simulink subsystem "matteEnergyBalance"  (R2024a)
settings: Solver=VariableStepAuto  StartTime=0.0  StopTime=3600*24  RelTol=1e-3
undefined symbols (not defined in the file): air_specific_heat_capacity, bath_area, matte_specific_heat_capacity, slag_matte_heat_transfer_coefficient
settings Model: DataDictionary=constants.sldd  EnableAccessToBaseWorkspace=off  DefaultTestHarness=matteEnergyBalance_Harness_Constants  Creator=eunice.duplessis  LastModifiedBy=jason.miskin

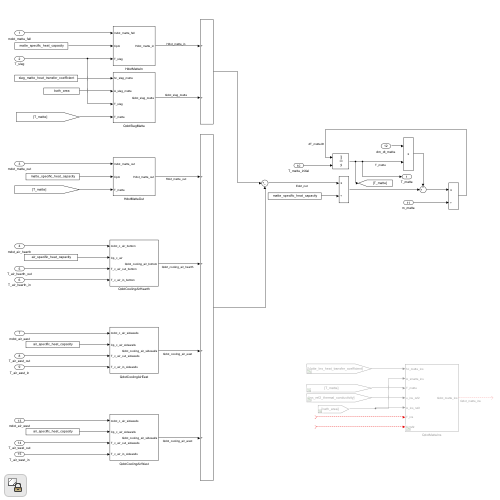
[thumbnail: Simulink's stored preview of the top-level diagram]
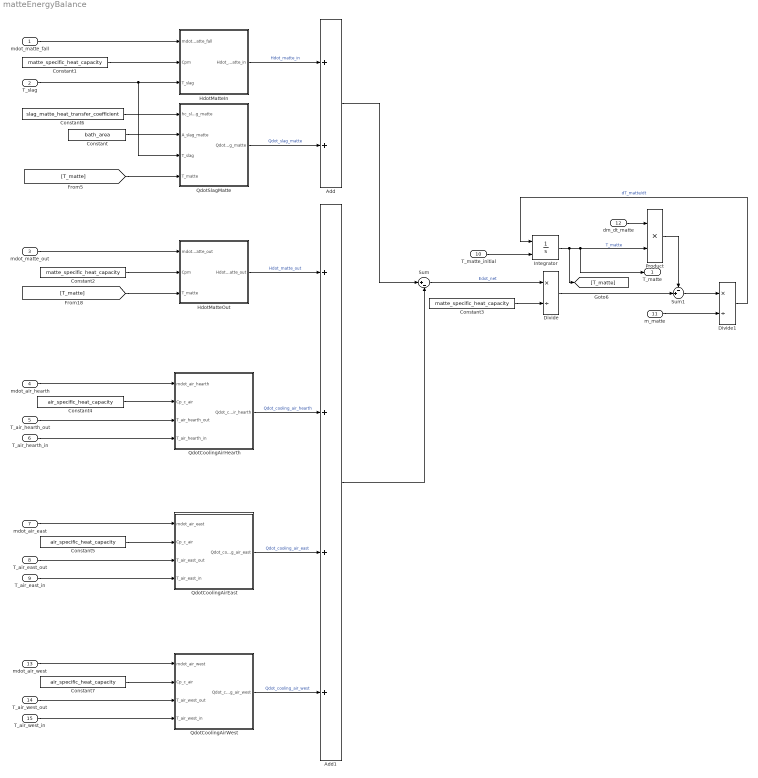
== system matteEnergyBalance ==
  mdot_matte_fall : Inport
  T_slag : Inport  Port=2
  mdot_matte_out : Inport  Port=3
  mdot_air_hearth : Inport  Port=4
  T_air_hearth_out : Inport  Port=5
  T_air_hearth_in : Inport  Port=6
  mdot_air_east : Inport  Port=7
  T_air_east_out : Inport  Port=8
  T_air_east_in : Inport  Port=9
  T_matte_initial : Inport  Port=10
  m_matte : Inport  Port=11
  dm_dt_matte : Inport  Port=12
  mdot_air_west : Inport  Port=13
  T_air_west_out : Inport  Port=14
  T_air_west_in : Inport  Port=15
  Add : Sum  Inputs=2
  Add1 : Sum  Inputs=4
  Constant : Constant  Value=bath_area
  Constant1 : Constant  Value=matte_specific_heat_capacity
  Constant2 : Constant  Value=matte_specific_heat_capacity
  Constant3 : Constant  Value=matte_specific_heat_capacity
  Constant4 : Constant  Value=air_specific_heat_capacity
  Constant5 : Constant  Value=air_specific_heat_capacity
  Constant6 : Constant  Value=slag_matte_heat_transfer_coefficient
  Constant7 : Constant  Value=air_specific_heat_capacity
  Divide : Product  Inputs=*/
  Divide1 : Product  Inputs=*/
  HdotMatteIn : Subsystem
  HdotMatteOut : Subsystem
  Integrator : Integrator  InitialConditionSource=external
  Product : Product
  QdotCoolingAirEast : Subsystem
  QdotCoolingAirHearth : Subsystem
  QdotCoolingAirWest : Subsystem
  QdotSlagMatte : Subsystem
  Sum : Sum  Inputs=|+-
  Sum1 : Sum  Inputs=-+|
  T_matte : Outport
  wires:
  Sum/1 -> Divide/1  "Edot_net"
  T_slag/1 -> QdotSlagMatte/3(T_slag), HdotMatteIn/3(T_slag)
  m_matte/1 -> Divide1/2
  [T_matte] -> QdotSlagMatte/4(T_matte)
  Product/1 -> Sum1/1
  dm_dt_matte/1 -> Product/1
  HdotMatteIn/1(Hdot_matte_in) -> Add/1  "Hdot_matte_in"
  Add/1 -> Sum/1
  Divide/1 -> Sum1/2
  Divide1/1 -> Integrator/1  "dT_matte/dt"
  Constant/1 -> QdotSlagMatte/2(A_slag_matte)
  Constant2/1 -> HdotMatteOut/2(Cpm)
  T_matte_initial/1 -> Integrator/2
  Integrator/1 -> [T_matte], T_matte/1, Product/2  "T_matte"
  HdotMatteOut/1(Hdot_matte_out) -> Add1/1  "Hdot_matte_out"
  mdot_air_east/1 -> QdotCoolingAirEast/1(mdot_air_east)
  mdot_matte_out/1 -> HdotMatteOut/1(mdot_matte_out)
  Sum1/1 -> Divide1/1
  QdotCoolingAirEast/1(Qdot_cooling_air_east) -> Add1/3  "Qdot_cooling_air_east"
  Constant6/1 -> QdotSlagMatte/1(hc_slag_matte)
  QdotSlagMatte/1(Qdot_slag_matte) -> Add/2  "Qdot_slag_matte"
  Constant3/1 -> Divide/2
  Constant1/1 -> HdotMatteIn/2(Cpm)
  Add1/1 -> Sum/2
  [T_matte] -> HdotMatteOut/3(T_matte)
  mdot_matte_fall/1 -> HdotMatteIn/1(mdot_matte_fall)
  Constant5/1 -> QdotCoolingAirEast/2(Cp_c_air)
  T_air_east_out/1 -> QdotCoolingAirEast/3(T_air_east_out)
  T_air_east_in/1 -> QdotCoolingAirEast/4(T_air_east_in)
  T_air_hearth_in/1 -> QdotCoolingAirHearth/4(T_air_hearth_in)
  Constant4/1 -> QdotCoolingAirHearth/2(Cp_c_air)
  QdotCoolingAirHearth/1(Qdot_cooling_air_hearth) -> Add1/2  "Qdot_cooling_air_hearth"
  mdot_air_hearth/1 -> QdotCoolingAirHearth/1(mdot_air_hearth)
  T_air_hearth_out/1 -> QdotCoolingAirHearth/3(T_air_hearth_out)
  T_air_west_in/1 -> QdotCoolingAirWest/4(T_air_west_in)
  T_air_west_out/1 -> QdotCoolingAirWest/3(T_air_west_out)
  Constant7/1 -> QdotCoolingAirWest/2(Cp_c_air)
  QdotCoolingAirWest/1(Qdot_cooling_air_west) -> Add1/4  "Qdot_cooling_air_west"
  mdot_air_west/1 -> QdotCoolingAirWest/1(mdot_air_west)

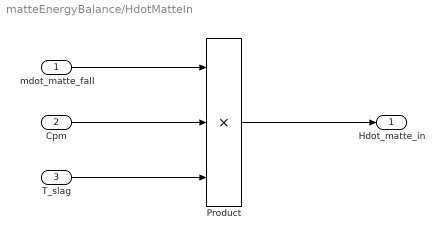
== system matteEnergyBalance/HdotMatteIn ==
  mdot_matte_fall : Inport
  Cpm : Inport  Port=2
  T_slag : Inport  Port=3
  Product : Product  Inputs=3
  Hdot_matte_in : Outport
  wires:
  T_slag/1 -> Product/3
  mdot_matte_fall/1 -> Product/1
  Product/1 -> Hdot_matte_in/1
  Cpm/1 -> Product/2

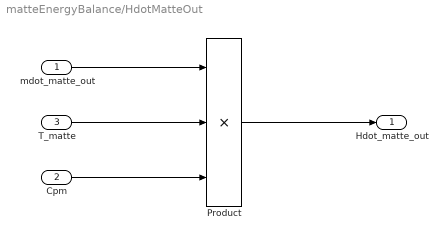
== system matteEnergyBalance/HdotMatteOut ==
  mdot_matte_out : Inport
  Cpm : Inport  Port=2
  T_matte : Inport  Port=3
  Product : Product  Inputs=3
  Hdot_matte_out : Outport
  wires:
  Cpm/1 -> Product/3
  mdot_matte_out/1 -> Product/1
  T_matte/1 -> Product/2
  Product/1 -> Hdot_matte_out/1

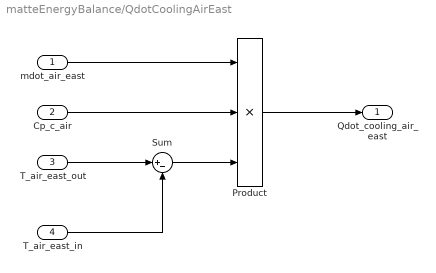
== system matteEnergyBalance/QdotCoolingAirEast ==
  mdot_air_east : Inport
  Cp_c_air : Inport  Port=2
  T_air_east_out : Inport  Port=3
  T_air_east_in : Inport  Port=4
  Product : Product  Inputs=3
  Sum : Sum  Inputs=|+-
  Qdot_cooling_air_east : Outport
  wires:
  mdot_air_east/1 -> Product/1
  T_air_east_out/1 -> Sum/1
  T_air_east_in/1 -> Sum/2
  Sum/1 -> Product/3
  Cp_c_air/1 -> Product/2
  Product/1 -> Qdot_cooling_air_east/1

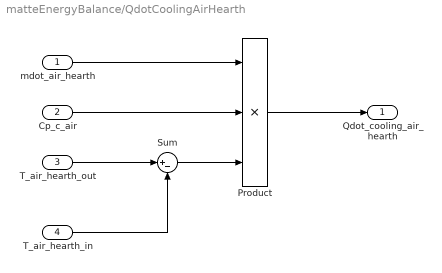
== system matteEnergyBalance/QdotCoolingAirHearth ==
  mdot_air_hearth : Inport
  Cp_c_air : Inport  Port=2
  T_air_hearth_out : Inport  Port=3
  T_air_hearth_in : Inport  Port=4
  Product : Product  Inputs=3
  Sum : Sum  Inputs=|+-
  Qdot_cooling_air_hearth : Outport
  wires:
  mdot_air_hearth/1 -> Product/1
  T_air_hearth_out/1 -> Sum/1
  T_air_hearth_in/1 -> Sum/2
  Sum/1 -> Product/3
  Cp_c_air/1 -> Product/2
  Product/1 -> Qdot_cooling_air_hearth/1

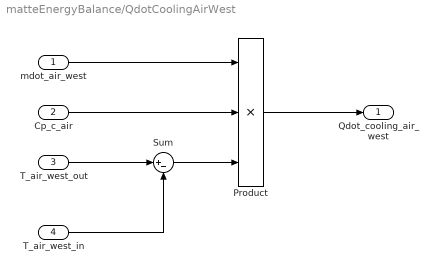
== system matteEnergyBalance/QdotCoolingAirWest ==
  mdot_air_west : Inport
  Cp_c_air : Inport  Port=2
  T_air_west_out : Inport  Port=3
  T_air_west_in : Inport  Port=4
  Product : Product  Inputs=3
  Sum : Sum  Inputs=|+-
  Qdot_cooling_air_west : Outport
  wires:
  Product/1 -> Qdot_cooling_air_west/1
  Cp_c_air/1 -> Product/2
  Sum/1 -> Product/3
  T_air_west_in/1 -> Sum/2
  T_air_west_out/1 -> Sum/1
  mdot_air_west/1 -> Product/1

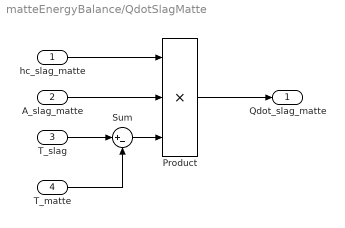
== system matteEnergyBalance/QdotSlagMatte ==
  hc_slag_matte : Inport
  A_slag_matte : Inport  Port=2
  T_slag : Inport  Port=3
  T_matte : Inport  Port=4
  Product : Product  Inputs=3
  Sum : Sum  Inputs=|+-
  Qdot_slag_matte : Outport
  wires:
  Product/1 -> Qdot_slag_matte/1
  Sum/1 -> Product/3
  T_matte/1 -> Sum/2
  T_slag/1 -> Sum/1
  A_slag_matte/1 -> Product/2
  hc_slag_matte/1 -> Product/1
